simulink model "leader_qball2_mytest"  (R2014a)
settings: Solver=ode1  StartTime=0.0  StopTime=inf  FixedStep=0.002  RelTol=1e-3
InitFcn:
  | QBall_2_Setup
values from neighbouring files (symbols this model uses):
  g = 9.81    [QBall_2_System_Parameters.m]
  joystick_range_max = 0.8    [QBall_2_Setup.m]
  joystick_range_min = 0.5    [QBall_2_Setup.m]
  KdHEIGHT_DOWN = 0.15    [QBall_2_Controller_Design.m]
  KdHEIGHT_UP = 0.15    [QBall_2_Controller_Design.m]
  KdOUTER_PITCH_DOWN = 0.4    [QBall_2_Controller_Design.m]
  KdOUTER_PITCH_UP = 0.6    [QBall_2_Controller_Design.m]
  KdOUTER_ROLL_DOWN = 0.4    [QBall_2_Controller_Design.m]
  KdOUTER_ROLL_UP = 0.4    [QBall_2_Controller_Design.m]
  KdPITCH_DOWN = 0.1    [QBall_2_Controller_Design.m]
  KdPITCH_UP = 0.1    [QBall_2_Controller_Design.m]
  KdROLL_DOWN = 0.1    [QBall_2_Controller_Design.m]
  KdROLL_UP = 0.1    [QBall_2_Controller_Design.m]
  KdYAW_DOWN = 0.32    [QBall_2_Controller_Design.m]
  KdYAW_UP = 0.32    [QBall_2_Controller_Design.m]
  KiHEIGHT_DOWN = 0.35    [QBall_2_Controller_Design.m]
  KiHEIGHT_UP = 0.35    [QBall_2_Controller_Design.m]
  KiOUTER_PITCH_DOWN = 0.08    [QBall_2_Controller_Design.m]
  KiOUTER_PITCH_UP = 0.08    [QBall_2_Controller_Design.m]
  KiOUTER_ROLL_DOWN = 0.08    [QBall_2_Controller_Design.m]
  KiOUTER_ROLL_UP = 0.08    [QBall_2_Controller_Design.m]
  KiPITCH_DOWN = 0.08    [QBall_2_Controller_Design.m]
  KiPITCH_UP = 0.08    [QBall_2_Controller_Design.m]
  KiROLL_DOWN = 0.08    [QBall_2_Controller_Design.m]
  KiROLL_UP = 0.08    [QBall_2_Controller_Design.m]
  KiYAW_DOWN = 0.0    (= 0)    [QBall_2_Controller_Design.m]
  KiYAW_UP = 0.0    (= 0)    [QBall_2_Controller_Design.m]
  KpHEIGHT_DOWN = 0.5    [QBall_2_Controller_Design.m]
  KpHEIGHT_UP = 0.5    [QBall_2_Controller_Design.m]
  KpOUTER_PITCH_DOWN = 0.3    [QBall_2_Controller_Design.m]
  KpOUTER_PITCH_UP = 0.3    [QBall_2_Controller_Design.m]
  KpOUTER_ROLL_DOWN = 0.3    [QBall_2_Controller_Design.m]
  KpOUTER_ROLL_UP = 0.3    [QBall_2_Controller_Design.m]
  KpPITCH_DOWN = 0.5    [QBall_2_Controller_Design.m]
  KpPITCH_UP = 0.5    [QBall_2_Controller_Design.m]
  KpROLL_DOWN = 0.5    [QBall_2_Controller_Design.m]
  KpROLL_UP = 0.5    [QBall_2_Controller_Design.m]
  KpYAW_DOWN = 0.45    [QBall_2_Controller_Design.m]
  KpYAW_UP = 0.45    [QBall_2_Controller_Design.m]
  LIMIT_CMD_PITCH = 5*pi/180    (= 0.0872664625997)    [QBall_2_Controller_Design.m]
  LIMIT_CMD_ROLL = 5*pi/180    (= 0.0872664625997)    [QBall_2_Controller_Design.m]
  LIMIT_MAX_HEIGHT = 2    [QBall_2_Controller_Design.m]
  LIMIT_MAX_X = 1    [QBall_2_Controller_Design.m]
  LIMIT_MAX_Z = 1    [QBall_2_Controller_Design.m]
  LIMIT_MIN_HEIGHT = 0.3    [QBall_2_Controller_Design.m]
  LIMIT_MIN_X = -1    [QBall_2_Controller_Design.m]
  LIMIT_MIN_Z = -1    [QBall_2_Controller_Design.m]
  LIMIT_RATE_HEIGHT = 0.05    [QBall_2_Controller_Design.m]
  LIMIT_RATE_X = 0.15    [QBall_2_Controller_Design.m]
  LIMIT_RATE_YAW = 15*pi/180    (= 0.261799387799)    [QBall_2_Controller_Design.m]
  LIMIT_RATE_Z = 0.15    [QBall_2_Controller_Design.m]
  LIMIT_uCMD_PITCH = 0.5    [QBall_2_Controller_Design.m]
  LIMIT_uCMD_ROLL = 0.5    [QBall_2_Controller_Design.m]
  LIMIT_uCMD_YAW = 0.5    [QBall_2_Controller_Design.m]
  OFFSET_HEIGHT = 0.3    [QBall_2_System_Parameters.m]
  OMEGA_FILTER = 60    [QBall_2_System_Parameters.m]
  TRIM_THROTTLE = M*g/(4*K)    [QBall_2_Controller_Design.m]
  TRIM_U_PITCH = 0.009    [QBall_2_Controller_Design.m]
  TRIM_U_ROLL = -0.0065    [QBall_2_Controller_Design.m]
undefined symbols (not defined in the file or in its folder): DiscIntNeverNeededParam, qc_get_step_size
libraries: simulink x27, quarc_library x27
(part 2 of 3)

== system leader_qball2_mytest/Throttle and height control/Joystick mode throttle ==
  Divide : Product  Inputs=**
  Joystick throttle scaling : Gain  Gain=0.8
  Joystick to Throttle Mapping : MATLAB Function  TreatAsAtomicUnit=on
  height command1 : Constant  Value=joystick_range_min
  height command2 : Constant  Value=joystick_range_max
  throttle joystick : Scope
      settings: YMin=0.45  YMax=1  SaveName=ScopeData26
  throttle : Outport
  wires:
  Divide/1 -> Joystick to Throttle Mapping/1(u)
  [throttle_joystick] -> throttle joystick/1, Divide/2
  [thrust_comp] -> Divide/1
  height command2/1 -> Joystick to Throttle Mapping/3(l2)
  height command1/1 -> Joystick to Throttle Mapping/2(l1)
  Joystick to Throttle Mapping/1(y) -> Joystick throttle scaling/1
  Joystick throttle scaling/1 -> throttle/1

== system leader_qball2_mytest/Throttle and height control/Safety - Active During Emergency Landing: Ramp Throttle CMD down to zero if Sonar Failed  ==
  note: The sonar is only used for an emergency landing if
      | the height mode is set to closed-loop. In joystick
      | height mode, the throttle wind down subsystem is
      | used to reduce the throttle to 0%.
  note: Check if the sonar value is changing.
      | If the sonar value does not change for 1 second
      | we assume the sonar is not connected or is malfunctioning,
      | in which case we want to reduce throttle quickly.
  throttle : Inport
  Limit descent rate : Subsystem
  Logical Operator : Logic  AllPortsSameDT=off  OutDataTypeStr=boolean
  Logical Operator1 : Logic  Operator=NOT  AllPortsSameDT=off  OutDataTypeStr=boolean
  Subsystem : Subsystem
  Switch : Switch  Threshold=0.5
  land w/ sonar : Scope
      settings: YMin=-0.2  YMax=1.2  SaveName=ScopeData25
  Out1 : Outport
  wires:
  Limit descent rate/1(throttle wind down) -> Switch/1
  Logical Operator/1 -> Switch/2
  Switch/1 -> Out1/1
  [land] -> Logical Operator/1, Limit descent rate/2(land)
  throttle/1 -> Switch/3, Limit descent rate/1(throttle)
  Subsystem/1(land with sonar) -> land w/ sonar/1, Logical Operator1/1
  Logical Operator1/1 -> Logical Operator/2

== system leader_qball2_mytest/Throttle and height control/height control ==
  height command : Inport
  Manual Switch : ManualSwitch  CurrentSetting=0
  Safety - Emergency Landing (Set Height Ref CMD to zero) : Subsystem
  Saturation3 : Saturate  UpperLimit=2  LowerLimit=0
  sigmoid1 : Subsystem
  sonar controller : Subsystem
  sonar height : Subsystem
  throttle : Outport
  tag scope: h_cmd=global
  wires:
  sonar controller/1(control_action) -> throttle/1
  sigmoid1/1(height_cmd) -> sonar controller/1(cmd), [h_cmd]
  sonar height/1(sonar (adjusted)) -> Saturation3/1
  Safety - Emergency Landing (Set Height Ref CMD to zero)/1(Out1) -> sigmoid1/1(cmd)
  height command/1 -> Safety - Emergency Landing (Set Height Ref CMD to zero)/1(In1)
  Saturation3/1 -> Manual Switch/1
  Manual Switch/1 -> sigmoid1/2(height), sonar controller/2(height)
  [height_above_ground] -> Manual Switch/2

== system leader_qball2_mytest/Control signal mixing/Safety - Motor Shutoff if: - Roll//Pitch Data Runaway (> 40 deg) - Initial 3 second of execution for motor initialization/Enabled Subsystem ==
  Enable : EnablePort
  Constant : Constant  Value=0
  Out1 : Outport  InitialOutput=1
  wires:
  Constant/1 -> Out1/1

== system leader_qball2_mytest/Control signal mixing/Safety - Motor Shutoff if: - Roll//Pitch Data Runaway (> 40 deg) - Initial 3 second of execution for motor initialization/throttle enable ==
  note: This check is obsolete - originally for protecting against invalid PWM command to ESC (for QBall-X4).
  Compare To Constant : simulink/Logic and Bit Operations/Compare To Constant  relop=<=  const=0.0525  OutDataTypeStr=uint8  ZeroCross=off
  Constant2 : Constant  Value=2
  Enabled Subsystem : Subsystem  TreatAsAtomicUnit=on
  Logical Operator1 : Logic  Operator=NOT  AllPortsSameDT=off  OutDataTypeStr=boolean
  en : Outport
  wires:
  [throttle_cmd] -> Compare To Constant/1
  Compare To Constant/1 -> Enabled Subsystem/Enable
  Enabled Subsystem/1(timeout) -> Logical Operator1/1
  Logical Operator1/1 -> en/1
  Constant2/1 -> Enabled Subsystem/1(timeout limit)

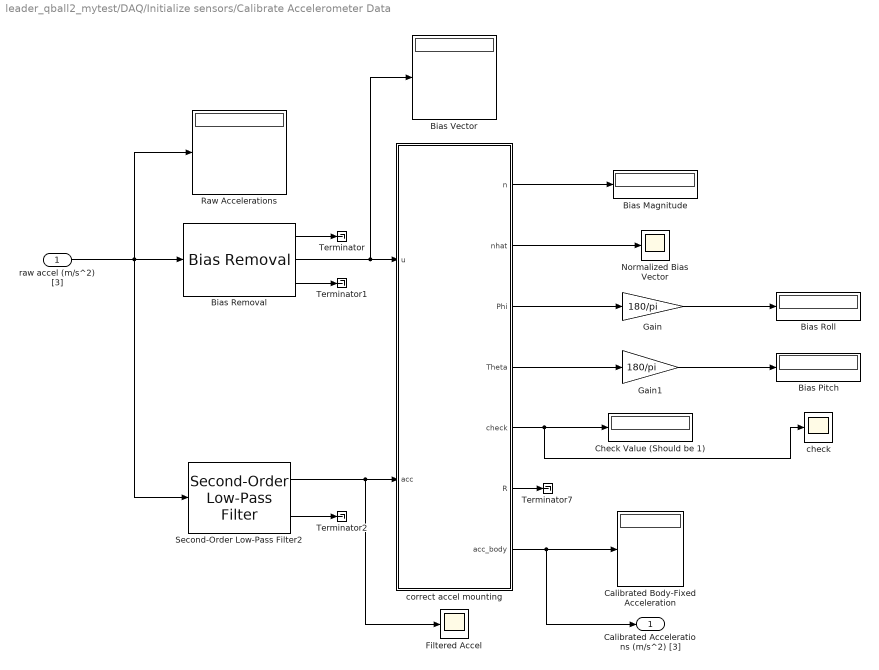
== system leader_qball2_mytest/DAQ/Initialize sensors/Calibrate Accelerometer Data ==
  raw accel (m/s^2) [3] : Inport
  Bias Magnitude : Display
      settings: Decimation=100
  Bias Pitch : Display
      settings: Decimation=100
  Bias Removal : quarc_library/Discrete/Bias Removal  start_time=0  end_time=TIMEOUT_CALIB  switch_id=0  sample_time=qc_get_step_size
  Bias Roll : Display
      settings: Decimation=100
  Bias Vector : Display
      settings: Decimation=100
  Calibrated Body-Fixed Acceleration : Display
      settings: Decimation=100
  Check Value (Should be 1) : Display
      settings: Decimation=100
  Filtered Accel : Scope
      settings: YMin=-200  YMax=200  SaveName=ScopeData42
  Gain : Gain  Gain=180/pi
  Gain1 : Gain  Gain=180/pi
  Normalized Bias Vector : Scope
  Raw Accelerations : Display
      settings: Decimation=100
  Second-Order Low-Pass Filter2 : quarc_library/Continuous/Second-Order Low-Pass Filter  params_source=Internal (dialog parameters)  input_width=OMEGA_FILTER  input_zeta=1  input_init=0
  Terminator{,1..2,7} (4 alike) : Terminator
  check : Scope
      settings: YMin=0.95  YMax=1.05  SaveName=ScopeData12
  correct accel mounting : MATLAB Function  TreatAsAtomicUnit=on
  Calibrated Accelerations (m/s^2) [3] : Outport
  wires:
  Bias Removal/2 -> Bias Vector/1, correct accel mounting/1(u)
  correct accel mounting/1(n) -> Bias Magnitude/1
  correct accel mounting/2(nhat) -> Normalized Bias Vector/1
  correct accel mounting/3(Phi) -> Gain/1
  correct accel mounting/4(Theta) -> Gain1/1
  Gain/1 -> Bias Roll/1
  Gain1/1 -> Bias Pitch/1
  correct accel mounting/5(check) -> check/1, Check Value (Should be 1)/1
  Bias Removal/1 -> Terminator/1
  Bias Removal/3 -> Terminator1/1
  correct accel mounting/6(R) -> Terminator7/1
  correct accel mounting/7(acc_body) -> Calibrated Accelerations (m/s^2) [3]/1, Calibrated Body-Fixed Acceleration/1
  raw accel (m/s^2) [3]/1 -> Raw Accelerations/1, Second-Order Low-Pass Filter2/1, Bias Removal/1
  Second-Order Low-Pass Filter2/1 -> Filtered Accel/1, correct accel mounting/2(acc)
  Second-Order Low-Pass Filter2/2 -> Terminator2/1

== system leader_qball2_mytest/DAQ/Initialize sensors/Calibrate accelerometer (Obsolete) ==
  In1 : Inport
  Calibration time (s) : Constant
  Clock : Clock
  Demux : Demux  Outputs=3
  Demux1 : Demux  Outputs=3
  Enabled Moving Average : quarc_library/Discrete/Enabled Moving Average  enable_state=reset  sample_time=qc_get_step_size
  Mux : Mux  Inputs=2
  Relational Operator : RelationalOperator  Operator=<  OutDataTypeStr=boolean
  Sum : Sum  Inputs=|+-
  Sum1 : Sum  Inputs=|+-
  Terminator{,1..3} (4 alike) : Terminator
  accel calibrated : Scope
      settings: YMin=-13  SaveName=ScopeData17
  accels offset : Scope
      settings: YMin=-13  SaveName=ScopeData16
  initial accel : Constant  Value=[0 0 -9.81]
  Out1 : Outport
  wires:
  In1/1 -> Sum1/1, Sum/1, Demux/1
  Clock/1 -> Relational Operator/1
  Calibration time (s)/1 -> Relational Operator/2
  Relational Operator/1 -> Enabled Moving Average/Enable
  Sum/1 -> Out1/1, Demux1/1
  initial accel/1 -> Sum1/2
  Sum1/1 -> Enabled Moving Average/1
  Enabled Moving Average/1 -> Sum/2, accels offset/1
  Demux/2 -> Mux/1
  Demux1/2 -> Mux/2
  Mux/1 -> accel calibrated/1
  Demux/1 -> Terminator/1
  Demux/3 -> Terminator1/1
  Demux1/1 -> Terminator2/1
  Demux1/3 -> Terminator3/1

== system leader_qball2_mytest/DAQ/Initialize sensors/Nonlinear Limit (Reject Spikes) ==
  u : Inport
  Constant : Constant  Value=0.5
  Embedded MATLAB Function : MATLAB Function  TreatAsAtomicUnit=on
  Memory : Memory
  y : Outport
  wires:
  Embedded MATLAB Function/1(y) -> Memory/1, y/1
  Memory/1 -> Embedded MATLAB Function/2(x)
  u/1 -> Embedded MATLAB Function/1(u)
  Constant/1 -> Embedded MATLAB Function/3(threshold)

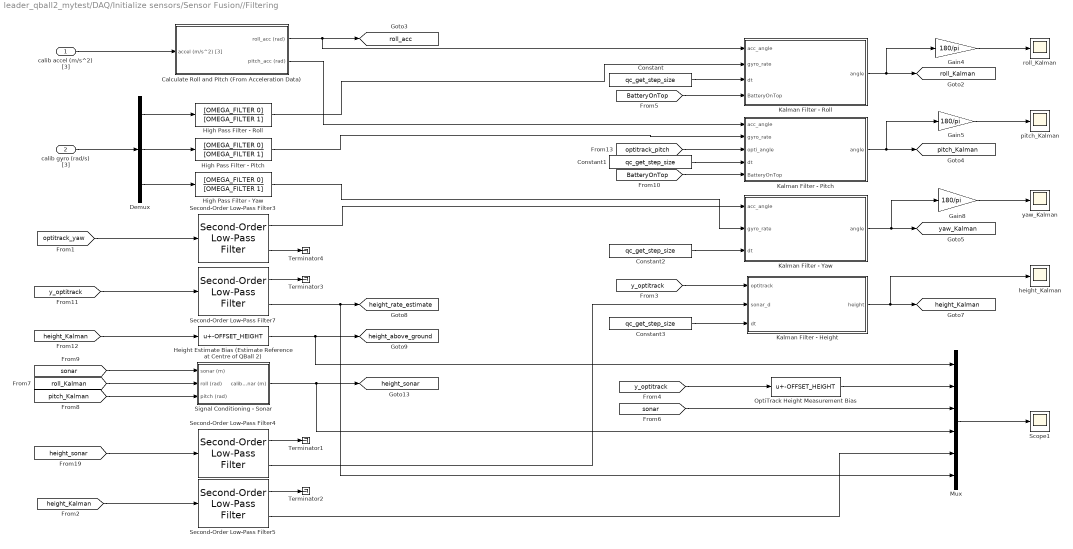
== system leader_qball2_mytest/DAQ/Initialize sensors/Sensor Fusion//Filtering ==
  calib accel (m/s^2) [3] : Inport
  calib gyro (rad/s) [3] : Inport  Port=2
  Calculate Roll and Pitch (From Acceleration Data) : Subsystem
  Constant{,1..3} (4 alike) : Constant  Value=qc_get_step_size
  Demux : Demux  Outputs=3
  Gain4 : Gain  Gain=180/pi
  Gain5 : Gain  Gain=180/pi
  Gain8 : Gain  Gain=180/pi
  "Height Estimate Bias (Estimate Reference at Centre of QBall 2) " : Bias  Bias=-OFFSET_HEIGHT
  High Pass Filter - Pitch : TransferFcn  Numerator=[OMEGA_FILTER 0]  Denominator=[OMEGA_FILTER 1]
  High Pass Filter - Roll : TransferFcn  Numerator=[OMEGA_FILTER 0]  Denominator=[OMEGA_FILTER 1]
  High Pass Filter - Yaw : TransferFcn  Numerator=[OMEGA_FILTER 0]  Denominator=[OMEGA_FILTER 1]
  Kalman Filter - Height : MATLAB Function  TreatAsAtomicUnit=on
  Kalman Filter - Pitch : MATLAB Function  TreatAsAtomicUnit=on
  Kalman Filter - Roll : MATLAB Function  TreatAsAtomicUnit=on
  Kalman Filter - Yaw : MATLAB Function  TreatAsAtomicUnit=on
  Mux : Mux  Inputs=6
  OptiTrack Height Measurement Bias : Bias  Bias=-OFFSET_HEIGHT
  Scope1 : Scope
      settings: YMin=-1.5  YMax=1.5  SaveName=ScopeData53
  Second-Order Low-Pass Filter3 : quarc_library/Continuous/Second-Order Low-Pass Filter  params_source=Internal (dialog parameters)  input_width=OMEGA_FILTER  input_zeta=1  input_init=0
  Second-Order Low-Pass Filter4 : quarc_library/Continuous/Second-Order Low-Pass Filter  params_source=Internal (dialog parameters)  input_width=OMEGA_DIFF  input_zeta=1  input_init=0
  Second-Order Low-Pass Filter5 : quarc_library/Continuous/Second-Order Low-Pass Filter  params_source=Internal (dialog parameters)  input_width=OMEGA_DIFF  input_zeta=1  input_init=0
  Second-Order Low-Pass Filter7 : quarc_library/Continuous/Second-Order Low-Pass Filter  params_source=Internal (dialog parameters)  input_width=OMEGA_DIFF  input_zeta=1  input_init=0
  Signal Conditioning - Sonar : Subsystem
  Terminator{1..4} (4 alike) : Terminator
  height_Kalman : Scope
      settings: YMin=17.282  YMax=17.292  SaveName=ScopeData52
  pitch_Kalman : Scope
      settings: TimeRange=10  YMin=-45  YMax=60  SaveName=ScopeData39
  roll_Kalman : Scope
      settings: YMin=-100  YMax=100  SaveName=ScopeData36
  yaw_Kalman : Scope
      settings: YMin=-70  YMax=110  SaveName=ScopeData47
  tag scope: height_Kalman=global, height_above_ground=global, height_rate_estimate=global, height_sonar=global, pitch_Kalman=global, roll_Kalman=global, roll_acc=global, yaw_Kalman=global
  wires:
  Kalman Filter - Roll/1(angle) -> [roll_Kalman], Gain4/1
  Demux/2 -> High Pass Filter - Pitch/1
  Constant/1 -> Kalman Filter - Roll/3(dt)
  Constant1/1 -> Kalman Filter - Pitch/4(dt)
  Kalman Filter - Pitch/1(angle) -> [pitch_Kalman], Gain5/1
  Gain5/1 -> pitch_Kalman/1
  Demux/3 -> High Pass Filter - Yaw/1
  Gain4/1 -> roll_Kalman/1
  calib gyro (rad/s) [3]/1 -> Demux/1
  Demux/1 -> High Pass Filter - Roll/1
  High Pass Filter - Roll/1 -> Kalman Filter - Roll/2(gyro_rate)
  [optitrack_yaw] -> Second-Order Low-Pass Filter3/1
  Second-Order Low-Pass Filter3/1 -> Kalman Filter - Yaw/1(acc_angle)
  High Pass Filter - Yaw/1 -> Kalman Filter - Yaw/2(gyro_rate)
  Constant2/1 -> Kalman Filter - Yaw/3(dt)
  Kalman Filter - Yaw/1(angle) -> [yaw_Kalman], Gain8/1
  Gain8/1 -> yaw_Kalman/1
  Constant3/1 -> Kalman Filter - Height/3(dt)
  Kalman Filter - Height/1(height) -> height_Kalman/1, [height_Kalman]
  Mux/1 -> Scope1/1
  Second-Order Low-Pass Filter4/2 -> Kalman Filter - Height/2(sonar_d)
  [y_optitrack] -> OptiTrack Height Measurement Bias/1
  [sonar] -> Mux/3
  OptiTrack Height Measurement Bias/1 -> Mux/2
  [y_optitrack] -> Kalman Filter - Height/1(optitrack)
  [height_Kalman] -> Second-Order Low-Pass Filter5/1
  Second-Order Low-Pass Filter5/2 -> Mux/5
  [y_optitrack] -> Second-Order Low-Pass Filter7/1
  Second-Order Low-Pass Filter7/2 -> Mux/6, [height_rate_estimate]
  [height_Kalman] -> "Height Estimate Bias (Estimate Reference at Centre of QBall 2) "/1
  "Height Estimate Bias (Estimate Reference at Centre of QBall 2) "/1 -> Mux/1, [height_above_ground]
  calib accel (m/s^2) [3]/1 -> Calculate Roll and Pitch (From Acceleration Data)/1(accel (m/s^2) [3])
  Calculate Roll and Pitch (From Acceleration Data)/1(roll_acc (rad)) -> Kalman Filter - Roll/1(acc_angle), [roll_acc]
  Calculate Roll and Pitch (From Acceleration Data)/2(pitch_acc (rad)) -> Kalman Filter - Pitch/1(acc_angle)
  Second-Order Low-Pass Filter3/2 -> Terminator4/1
  Second-Order Low-Pass Filter7/1 -> Terminator3/1
  [roll_Kalman] -> Signal Conditioning - Sonar/2(roll (rad))
  [pitch_Kalman] -> Signal Conditioning - Sonar/3(pitch (rad))
  [sonar] -> Signal Conditioning - Sonar/1(sonar (m))
  Signal Conditioning - Sonar/1(calib sonar (m)) -> Mux/4, [height_sonar]
  [height_sonar] -> Second-Order Low-Pass Filter4/1
  Second-Order Low-Pass Filter4/1 -> Terminator1/1
  Second-Order Low-Pass Filter5/1 -> Terminator2/1
  High Pass Filter - Pitch/1 -> Kalman Filter - Pitch/2(gyro_rate)
  [BatteryOnTop] -> Kalman Filter - Roll/4(BatteryOnTop)
  [BatteryOnTop] -> Kalman Filter - Pitch/5(BatteryOnTop)
  [optitrack_pitch] -> Kalman Filter - Pitch/3(opti_angle)

== system leader_qball2_mytest/DAQ/Initialize sensors/Zero gyro ==
  In1 : Inport
  Calibration time (s) : Constant
  Clock : Clock
  Enabled Moving Average : quarc_library/Discrete/Enabled Moving Average  enable_state=reset  sample_time=qc_get_step_size
  Relational Operator : RelationalOperator  Operator=<  OutDataTypeStr=boolean
  Sum : Sum  Inputs=|+-
  Out1 : Outport
  wires:
  Sum/1 -> Out1/1
  Relational Operator/1 -> Enabled Moving Average/Enable
  Calibration time (s)/1 -> Relational Operator/2
  Clock/1 -> Relational Operator/1
  Enabled Moving Average/1 -> Sum/2
  In1/1 -> Sum/1, Enabled Moving Average/1

== system leader_qball2_mytest/Data from host/rcvd packet monitoring/spike detection ==
  In1 : Inport
  Abs : Abs
  Compare To Constant : simulink/Logic and Bit Operations/Compare To Constant  relop=>=  const=100  OutDataTypeStr=boolean  ZeroCross=off
  Logical Operator4 : Logic  Operator=OR  Inputs=1  AllPortsSameDT=off  OutDataTypeStr=boolean
  Show Message on Host1 : quarc_library/Sinks/Error Handling/Show Message on Host  message_type=Fixed error message  message_icon=Warning  message=Spike detected!
      settings: AttributesFormatString="\"%<message>\""
  wires:
  Abs/1 -> Compare To Constant/1
  Compare To Constant/1 -> Logical Operator4/1
  Logical Operator4/1 -> Show Message on Host1/1
  In1/1 -> Abs/1

== system leader_qball2_mytest/Data from host/timeout safety/Enabled Subsystem ==
  timeout limit : Inport
  Enable : EnablePort  StatesWhenEnabling=reset
  Constant : Constant  SampleTime=qc_get_step_size
  Discrete-Time Integrator : DiscreteIntegrator  SampleTime=-1  ICPrevOutput=DiscIntNeverNeededParam  ICPrevScaledInput=DiscIntNeverNeededParam
  Relational Operator : RelationalOperator  OutDataTypeStr=boolean
  timeout : Outport  OutputWhenDisabled=reset  InitialOutput=[0]
  wires:
  Relational Operator/1 -> timeout/1
  timeout limit/1 -> Relational Operator/2
  Discrete-Time Integrator/1 -> Relational Operator/1
  Constant/1 -> Discrete-Time Integrator/1

== system leader_qball2_mytest/Data from host/timeout safety/Enabled Subsystem1 ==
  timeout limit : Inport
  Enable : EnablePort  StatesWhenEnabling=reset
  Constant : Constant  SampleTime=qc_get_step_size
  Discrete-Time Integrator : DiscreteIntegrator  SampleTime=-1  ICPrevOutput=DiscIntNeverNeededParam  ICPrevScaledInput=DiscIntNeverNeededParam
  Relational Operator : RelationalOperator  OutDataTypeStr=boolean
  timeout : Outport  OutputWhenDisabled=reset  InitialOutput=[0]
  wires:
  Relational Operator/1 -> timeout/1
  timeout limit/1 -> Relational Operator/2
  Discrete-Time Integrator/1 -> Relational Operator/1
  Constant/1 -> Discrete-Time Integrator/1

== system leader_qball2_mytest/Data from host/timeout safety/Enabled Subsystem2 ==
  Enable : EnablePort
  Constant : Constant
  Out1 : Outport  InitialOutput=0
  wires:
  Constant/1 -> Out1/1

== system leader_qball2_mytest/Data from host/timeout safety/Enabled Subsystem Latch Output High ==
  Enable : EnablePort
  Constant : Constant
  Out1 : Outport  InitialOutput=0
  wires:
  Constant/1 -> Out1/1

== system leader_qball2_mytest/Pitch Controller/Subsystem/OT pos control ==
  Compare To Constant : simulink/Logic and Bit Operations/Compare To Constant  relop=>  const=0.4*0  OutDataTypeStr=uint8  ZeroCross=off
  Mux1 : Mux  Inputs=2
  Orig v. adjusted pitch : Scope
      settings: YMin=-0.1  YMax=0.12  SaveName=ScopeData21
  Product : Product  RndMeth=Zero
  Sum2 : Sum  Inputs=+-
  adjust_for_heading : Subsystem
  rate limitted control : Subsystem
  pitch cmd : Outport
  tag scope: pitch_workspace_frame=global
  wires:
  rate limitted control/1(Pitch Ref CMD (rad)) -> Product/1, [pitch_workspace_frame]
  Sum2/1 -> rate limitted control/1(error)
  Product/1 -> Mux1/1, adjust_for_heading/1(original)
  Compare To Constant/1 -> Product/2
  [y_optitrack] -> Compare To Constant/1
  Mux1/1 -> Orig v. adjusted pitch/1
  adjust_for_heading/1(heading_adjusted pitch) -> Mux1/2, pitch cmd/1
  [z_optitrack] -> Sum2/2
  [z_pos_cmd] -> Sum2/1

== system leader_qball2_mytest/Pitch Controller/Subsystem/Safety - Emergency Landing Zero Ref CMD ==
  In1 : Inport
  Constant : Constant  Value=0
  Enabled Subsystem : Subsystem  TreatAsAtomicUnit=on
  Switch : Switch  Threshold=0.5
  Out1 : Outport
  wires:
  [land] -> Enabled Subsystem/Enable
  Constant/1 -> Switch/1
  Enabled Subsystem/1(Out1) -> Switch/2
  In1/1 -> Switch/3
  Switch/1 -> Out1/1

== system leader_qball2_mytest/Roll Controller/Subsystem/OT pos control ==
  Compare To Constant : simulink/Logic and Bit Operations/Compare To Constant  relop=>  const=0.4*0  OutDataTypeStr=uint8  ZeroCross=off
  Mux1 : Mux  Inputs=2
  Mux2 : Mux  Inputs=2
  Orig v. adjusted roll : Scope
      settings: YMin=-0.12  YMax=0.09  SaveName=ScopeData22
  Product : Product  RndMeth=Zero
  Sum1 : Sum  Inputs=+-
  X_cmd and X_meas : Scope
      settings: YMin=0  YMax=0.11  SaveName=ScopeData11
  adjust_for_heading : Subsystem
  rate limitted control : Subsystem
  roll cmd : Outport
  tag scope: roll_workspace_frame=global
  wires:
  rate limitted control/1(Roll Ref CMD (rad)) -> Product/1, [roll_workspace_frame]
  Sum1/1 -> rate limitted control/1(error)
  Product/1 -> Mux1/1, adjust_for_heading/1(original)
  Compare To Constant/1 -> Product/2
  [y_optitrack] -> Compare To Constant/1
  Mux1/1 -> Orig v. adjusted roll/1
  adjust_for_heading/1(heading_adjusted roll) -> Mux1/2, roll cmd/1
  [x_optitrack] -> Sum1/2, Mux2/2
  [x_pos_cmd] -> Sum1/1, Mux2/1
  Mux2/1 -> X_cmd and X_meas/1

== system leader_qball2_mytest/Roll Controller/Subsystem/Safety - Emergency Landing Zero Ref CMD ==
  In1 : Inport
  Constant : Constant  Value=0
  Enabled Subsystem : Subsystem  TreatAsAtomicUnit=on
  Switch : Switch  Threshold=0.5
  Out1 : Outport
  wires:
  Switch/1 -> Out1/1
  In1/1 -> Switch/3
  Enabled Subsystem/1(Out1) -> Switch/2
  Constant/1 -> Switch/1
  [land] -> Enabled Subsystem/Enable

== system leader_qball2_mytest/Throttle and height control/Safety - Active During Emergency Landing: Ramp Throttle CMD down to zero if Sonar Failed /Limit descent rate ==
  throttle : Inport
  land : Inport  Port=2
  Constant1 : Constant  Value=0
  Terminator : Terminator
  Terminator1 : Terminator
  Terminator2 : Terminator
  Triggered Sigmoid : quarc_library/Sources/Sigmoids/Triggered Sigmoid  params_source=Internal (dialog parameters)  max_velocity=0.04  max_acceleration=1000*20  hold_off=0.5  output_sample_time=qc_get_step_size  trigger=rising
  land throttle target : Constant  Value=0
  throttle wind down : Outport
  wires:
  Triggered Sigmoid/1 -> throttle wind down/1
  land throttle target/1 -> Triggered Sigmoid/4
  Constant1/1 -> Triggered Sigmoid/3
  throttle/1 -> Triggered Sigmoid/2
  land/1 -> Triggered Sigmoid/1
  Triggered Sigmoid/2 -> Terminator/1
  Triggered Sigmoid/3 -> Terminator1/1
  Triggered Sigmoid/4 -> Terminator2/1

== system leader_qball2_mytest/Throttle and height control/Safety - Active During Emergency Landing: Ramp Throttle CMD down to zero if Sonar Failed /Subsystem ==
  Compare To Constant : simulink/Logic and Bit Operations/Compare To Constant  relop===  const=1  OutDataTypeStr=uint8
  Compare To Zero : simulink/Logic and Bit Operations/Compare To Zero  relop===  OutDataTypeStr=boolean  ZeroCross=off
  Constant1 : Constant  Value=0
  Constant2 : Constant  Value=5
  Derivative : Derivative
  Enabled Subsystem1 : Subsystem  TreatAsAtomicUnit=on
  Logical Operator : Logic  AllPortsSameDT=off  OutDataTypeStr=boolean
  Logical Operator3 : Logic  Operator=NOT  AllPortsSameDT=off  OutDataTypeStr=boolean
  Manual Switch : ManualSwitch
  land with sonar : Outport
  wires:
  Logical Operator3/1 -> Logical Operator/1
  Compare To Constant/1 -> Logical Operator/2
  [height_mode] -> Compare To Constant/1
  Logical Operator/1 -> land with sonar/1
  Enabled Subsystem1/1(timeout) -> Logical Operator3/1
  Constant1/1 -> Manual Switch/2
  [sonar] -> Manual Switch/1
  Manual Switch/1 -> Derivative/1
  Constant2/1 -> Enabled Subsystem1/1(timeout limit)
  Compare To Zero/1 -> Enabled Subsystem1/Enable
  Derivative/1 -> Compare To Zero/1

== system leader_qball2_mytest/Throttle and height control/height control/Safety - Emergency Landing (Set Height Ref CMD to zero) ==
  In1 : Inport
  Constant : Constant  Value=0
  Enabled Subsystem : Subsystem  TreatAsAtomicUnit=on
  Switch : Switch  Threshold=0.5
  Out1 : Outport
  wires:
  Constant/1 -> Switch/1
  [land] -> Enabled Subsystem/Enable
  Enabled Subsystem/1(Out1) -> Switch/2
  In1/1 -> Switch/3
  Switch/1 -> Out1/1

== system leader_qball2_mytest/Throttle and height control/height control/sigmoid1 ==
  cmd : Inport
  height : Inport  Port=2
  Continuous Sigmoid : quarc_library/Sources/Sigmoids/Continuous Sigmoid  params_source=External (input ports)  max_velocity=2  max_acceleration=10  initial_position=0  initial_velocity=0  hold_off=0.5  input_sample_time=-1  output_sample_time=qc_get_step_size
  Terminator : Terminator
  Terminator1 : Terminator
  Terminator2 : Terminator
  arm height command : Subsystem  TreatAsAtomicUnit=on
  sigmoid limits : Subsystem
  height_cmd : Outport
  wires:
  Continuous Sigmoid/4 -> Terminator2/1
  Continuous Sigmoid/3 -> Terminator1/1
  Continuous Sigmoid/2 -> Terminator/1
  arm height command/1(Out1) -> Continuous Sigmoid/1
  cmd/1 -> arm height command/1(In1), sigmoid limits/1(height cmd)
  sigmoid limits/1(vmax) -> Continuous Sigmoid/2
  sigmoid limits/2(amax) -> Continuous Sigmoid/3
  [armed] -> arm height command/Enable
  height/1 -> sigmoid limits/2(height)
  Continuous Sigmoid/1 -> height_cmd/1

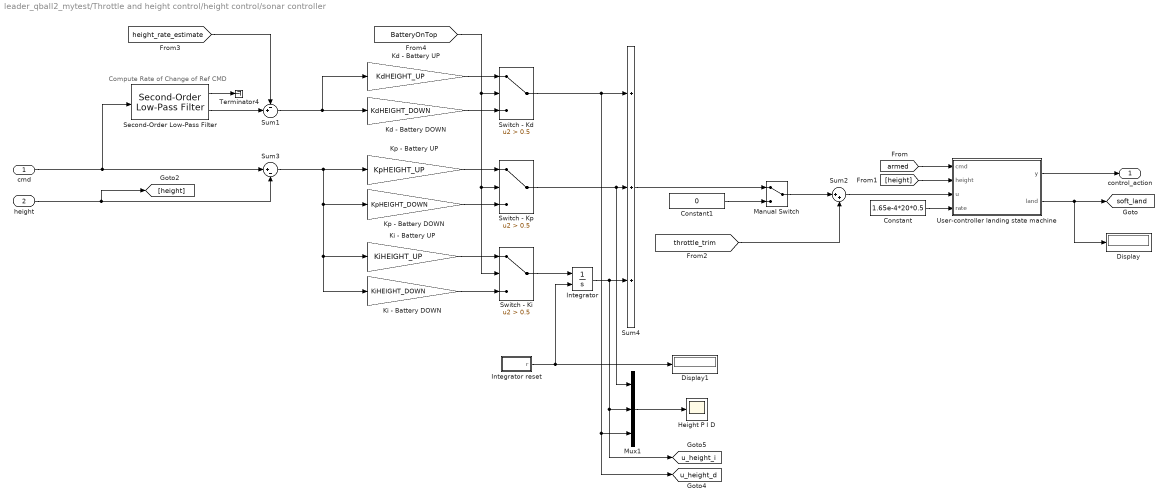
== system leader_qball2_mytest/Throttle and height control/height control/sonar controller ==
  note: Compute Rate of Change of Ref CMD
  cmd : Inport
  height : Inport  Port=2
  Constant : Constant  Value=1.65e-4*20*0.5
  Constant1 : Constant  Value=0
  Display : Display
      settings: Decimation=100
  Display1 : Display
      settings: Decimation=100
  Height P I D : Scope
      settings: YMin=-0.065  YMax=0.04  SaveName=ScopeData37
  Integrator : Integrator  ExternalReset=level  LimitOutput=on  UpperSaturationLimit=1  LowerSaturationLimit=0
  Integrator reset : Subsystem
  Kd - Battery DOWN : Gain  Gain=KdHEIGHT_DOWN
  Kd - Battery UP : Gain  Gain=KdHEIGHT_UP
  Ki - Battery DOWN : Gain  Gain=KiHEIGHT_DOWN
  Ki - Battery UP : Gain  Gain=KiHEIGHT_UP
  Kp - Battery DOWN : Gain  Gain=KpHEIGHT_DOWN
  Kp - Battery UP : Gain  Gain=KpHEIGHT_UP
  Manual Switch : ManualSwitch
  Mux1 : Mux  Inputs=3
  Second-Order Low-Pass Filter : quarc_library/Continuous/Second-Order Low-Pass Filter  params_source=Internal (dialog parameters)  input_width=OMEGA_DIFF  input_zeta=1  input_init=0
  Sum1 : Sum  Inputs=-+|
  Sum2 : Sum  Inputs=|++
  Sum3 : Sum  Inputs=|+-
  Sum4 : Sum  Inputs=+++
  Switch - Kd : Switch  Criteria=u2 > Threshold  Threshold=0.5
  Switch - Ki : Switch  Criteria=u2 > Threshold  Threshold=0.5
  Switch - Kp : Switch  Criteria=u2 > Threshold  Threshold=0.5
  Terminator4 : Terminator
  User-controller landing state machine : MATLAB Function  TreatAsAtomicUnit=on
  control_action : Outport
  tag scope: soft_land=global, u_height_d=global, u_height_i=global
  wires:
  Constant/1 -> User-controller landing state machine/4(rate)
  User-controller landing state machine/2(land) -> [soft_land], Display/1
  [height] -> User-controller landing state machine/2(height)
  [armed] -> User-controller landing state machine/1(cmd)
  User-controller landing state machine/1(y) -> control_action/1
  Mux1/1 -> Height P I D/1
  height/1 -> Sum3/2, [height]
  cmd/1 -> Sum3/1, Second-Order Low-Pass Filter/1
  Sum3/1 -> Kp - Battery UP/1, Ki - Battery UP/1, Ki - Battery DOWN/1, Kp - Battery DOWN/1
  Integrator reset/1(r) -> Display1/1, Integrator/2
  Integrator/1 -> [u_height_i], Mux1/2, Sum4/3
  Sum1/1 -> Kd - Battery DOWN/1, Kd - Battery UP/1
  Sum4/1 -> Manual Switch/1
  Constant1/1 -> Manual Switch/2
  Manual Switch/1 -> Sum2/1
  [throttle_trim] -> Sum2/2
  Sum2/1 -> User-controller landing state machine/3(u)
  Second-Order Low-Pass Filter/1 -> Terminator4/1
  Kd - Battery UP/1 -> Switch - Kd/1
  Kd - Battery DOWN/1 -> Switch - Kd/3
  [BatteryOnTop] -> Switch - Kp/2, Switch - Ki/2, Switch - Kd/2
  Switch - Kd/1 -> Mux1/3, [u_height_d], Sum4/1
  Kp - Battery UP/1 -> Switch - Kp/1
  Kp - Battery DOWN/1 -> Switch - Kp/3
  Switch - Kp/1 -> Mux1/1, Sum4/2
  [height_rate_estimate] -> Sum1/1
  Second-Order Low-Pass Filter/2 -> Sum1/2
  Ki - Battery DOWN/1 -> Switch - Ki/3
  Switch - Ki/1 -> Integrator/1
  Ki - Battery UP/1 -> Switch - Ki/1

== system leader_qball2_mytest/Throttle and height control/height control/sonar height ==
  Product : Product  Inputs=3  RndMeth=Zero
  Trigonometric Function : Trigonometry  Operator=cos
  Trigonometric Function2 : Trigonometry  Operator=cos
  sonar (adjusted) : Outport
  wires:
  Trigonometric Function2/1 -> Product/1
  [pitch_Kalman] -> Trigonometric Function2/1
  Trigonometric Function/1 -> Product/2
  Product/1 -> sonar (adjusted)/1
  [roll_Kalman] -> Trigonometric Function/1
  [sonar] -> Product/3

== system leader_qball2_mytest/Control signal mixing/Safety - Motor Shutoff if: - Roll//Pitch Data Runaway (> 40 deg) - Initial 3 second of execution for motor initialization/throttle enable/Enabled Subsystem ==
  timeout limit : Inport
  Enable : EnablePort  StatesWhenEnabling=reset
  Constant : Constant  SampleTime=qc_get_step_size
  Discrete-Time Integrator : DiscreteIntegrator  SampleTime=-1  ICPrevOutput=DiscIntNeverNeededParam  ICPrevScaledInput=DiscIntNeverNeededParam
  Relational Operator : RelationalOperator  OutDataTypeStr=boolean
  timeout : Outport  OutputWhenDisabled=reset  InitialOutput=[0]
  wires:
  Constant/1 -> Discrete-Time Integrator/1
  Discrete-Time Integrator/1 -> Relational Operator/1
  timeout limit/1 -> Relational Operator/2
  Relational Operator/1 -> timeout/1

== system leader_qball2_mytest/DAQ/Initialize sensors/Sensor Fusion//Filtering/Calculate Roll and Pitch (From Acceleration Data) ==
  accel (m/s^2) [3] : Inport
  Gain{1..2,6..7} (4 alike) : Gain  Gain=180/pi
  calc_roll_pitch : MATLAB Function  TreatAsAtomicUnit=on
  calc_roll_pitch_asin : MATLAB Function  TreatAsAtomicUnit=on
  pitch_acc : Scope
      settings: YMin=-60  YMax=45  SaveName=ScopeData28
  pitch_acc_asin : Scope
      settings: YMin=-10  YMax=27.5  SaveName=ScopeData43
  roll_acc : Scope
      settings: YMin=-200  YMax=200  SaveName=ScopeData20
  roll_acc_asin : Scope
      settings: TimeRange=10  YMin=-10  YMax=27.5  SaveName=ScopeData29
  roll_acc (rad) : Outport
  pitch_acc (rad) : Outport  Port=2
  wires:
  accel (m/s^2) [3]/1 -> calc_roll_pitch_asin/1(acc_body), calc_roll_pitch/1(acc_body)
  calc_roll_pitch/1(roll_acc) -> Gain2/1, roll_acc (rad)/1
  calc_roll_pitch/2(pitch_acc) -> Gain1/1, pitch_acc (rad)/1
  Gain2/1 -> roll_acc/1
  Gain1/1 -> pitch_acc/1
  calc_roll_pitch_asin/1(roll_acc) -> Gain6/1
  Gain6/1 -> roll_acc_asin/1
  calc_roll_pitch_asin/2(pitch_acc) -> Gain7/1
  Gain7/1 -> pitch_acc_asin/1

== system leader_qball2_mytest/DAQ/Initialize sensors/Sensor Fusion//Filtering/Signal Conditioning - Sonar ==
  note: Correct for Roll and Pitch
  note: "Smooth" out the Sonar data
  note: Resample the 10Hz Sonar Data
  sonar (m) : Inport
  roll (rad) : Inport  Port=2
  pitch (rad) : Inport  Port=3
  FOH1 : Subsystem  mask{Ts=0.1}
      mask prompts: Ts "Sample Time"
  Product : Product  Inputs=3  RndMeth=Zero
  Rate Transition : RateTransition
  Sampler : Subsystem  mask{Ts=0.1}
      mask prompts: Ts "Sample Time"
  Trigonometric Function : Trigonometry  Operator=cos
  Trigonometric Function2 : Trigonometry  Operator=cos
  calib sonar (m) : Outport
  wires:
  Sampler/1(Out1) -> Rate Transition/1
  Rate Transition/1 -> FOH1/1(Input)
  sonar (m)/1 -> Sampler/1(In1)
  FOH1/1(Output) -> Product/1
  Trigonometric Function2/1 -> Product/2
  roll (rad)/1 -> Trigonometric Function2/1
  pitch (rad)/1 -> Trigonometric Function/1
  Trigonometric Function/1 -> Product/3
  Product/1 -> calib sonar (m)/1

== system leader_qball2_mytest/Pitch Controller/Subsystem/OT pos control/adjust_for_heading ==
  original : Inport
  Memory : Memory
  adjust_pitch_command : MATLAB Function  TreatAsAtomicUnit=on
  heading_adjusted pitch : Outport
  wires:
  [heading_obs] -> adjust_pitch_command/3(heading)
  adjust_pitch_command/1(adj_pitch_cmd) -> Memory/1
  [roll_workspace_frame] -> adjust_pitch_command/2(roll_cmd)
  original/1 -> adjust_pitch_command/1(pitch_cmd)
  Memory/1 -> heading_adjusted pitch/1

== system leader_qball2_mytest/Pitch Controller/Subsystem/OT pos control/rate limitted control ==
  error : Inport
  Gain4 : Gain  Gain=-1
  Integrator : Integrator  ExternalReset=level
  Integrator reset : Subsystem
  Ki - Battery DOWN : Gain  Gain=KiOUTER_PITCH_DOWN
  Ki - Battery UP : Gain  Gain=KiOUTER_PITCH_UP
  Kp - Battery DOWN : Gain  Gain=KpOUTER_PITCH_DOWN
  Kp - Battery UP : Gain  Gain=KpOUTER_PITCH_UP
  Kv - Battery DOWN : Gain  Gain=KdOUTER_PITCH_DOWN
  Kv - Battery UP : Gain  Gain=KdOUTER_PITCH_UP
  Saturation1 : Saturate  UpperLimit=LIMIT_CMD_PITCH  LowerLimit=-LIMIT_CMD_PITCH
  Second-Order Low-Pass Filter1 : quarc_library/Continuous/Second-Order Low-Pass Filter  params_source=Internal (dialog parameters)  input_width=OMEGA_DIFF  input_zeta=1  input_init=0
  Sum4 : Sum  Inputs=-++
  Switch - Kd : Switch  Criteria=u2 > Threshold  Threshold=0.5
  Switch - Ki : Switch  Criteria=u2 > Threshold  Threshold=0.5
  Switch - Kp : Switch  Criteria=u2 > Threshold  Threshold=0.5
  Terminator4 : Terminator
  Pitch Ref CMD (rad) : Outport
  wires:
  Gain4/1 -> Pitch Ref CMD (rad)/1
  Saturation1/1 -> Gain4/1
  error/1 -> Kp - Battery UP/1, Ki - Battery UP/1, Ki - Battery DOWN/1, Kp - Battery DOWN/1
  Sum4/1 -> Saturation1/1
  Second-Order Low-Pass Filter1/2 -> Kv - Battery UP/1, Kv - Battery DOWN/1
  Integrator/1 -> Sum4/3
  [z_optitrack] -> Second-Order Low-Pass Filter1/1
  Integrator reset/1(r) -> Integrator/2
  Second-Order Low-Pass Filter1/1 -> Terminator4/1
  Kv - Battery DOWN/1 -> Switch - Kd/3
  Kv - Battery UP/1 -> Switch - Kd/1
  [BatteryOnTop] -> Switch - Kd/2, Switch - Kp/2, Switch - Ki/2
  Switch - Kd/1 -> Sum4/1
  Switch - Kp/1 -> Sum4/2
  Kp - Battery UP/1 -> Switch - Kp/1
  Kp - Battery DOWN/1 -> Switch - Kp/3
  Ki - Battery UP/1 -> Switch - Ki/1
  Ki - Battery DOWN/1 -> Switch - Ki/3
  Switch - Ki/1 -> Integrator/1

== system leader_qball2_mytest/Pitch Controller/Subsystem/Safety - Emergency Landing Zero Ref CMD/Enabled Subsystem ==
  Enable : EnablePort
  Constant : Constant
  Out1 : Outport  InitialOutput=0
  wires:
  Constant/1 -> Out1/1

== system leader_qball2_mytest/Roll Controller/Subsystem/OT pos control/adjust_for_heading ==
  original : Inport
  Memory : Memory
  adjust_roll_command : MATLAB Function  TreatAsAtomicUnit=on
  heading_adjusted roll : Outport
  wires:
  [heading_obs] -> adjust_roll_command/3(heading)
  [pitch_workspace_frame] -> adjust_roll_command/2(pitch_cmd)
  original/1 -> adjust_roll_command/1(roll_cmd)
  adjust_roll_command/1(adj_roll_cmd) -> Memory/1
  Memory/1 -> heading_adjusted roll/1

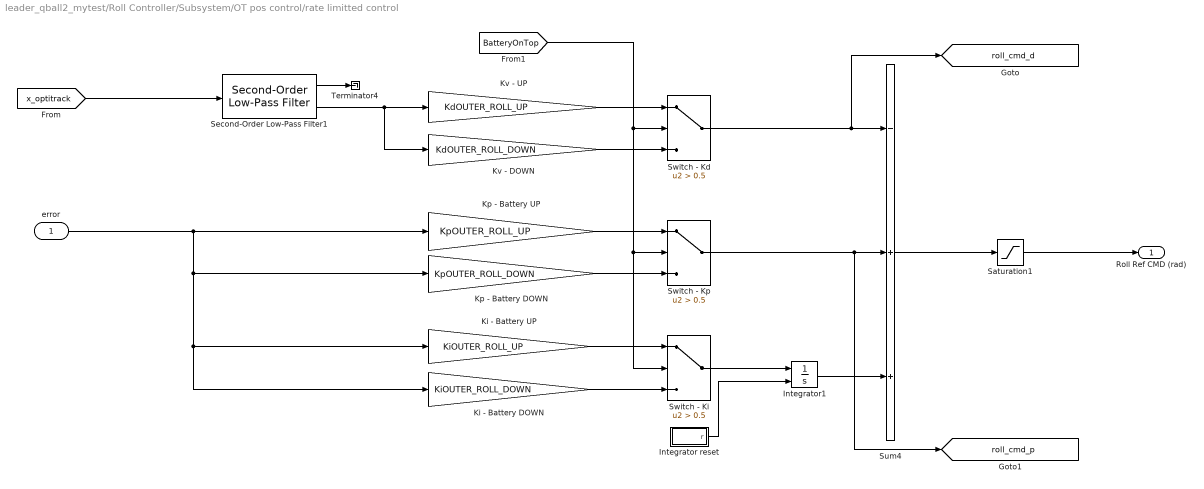
== system leader_qball2_mytest/Roll Controller/Subsystem/OT pos control/rate limitted control ==
  error : Inport
  Integrator reset : Subsystem
  Integrator1 : Integrator  ExternalReset=level
  Ki - Battery DOWN : Gain  Gain=KiOUTER_ROLL_DOWN
  Ki - Battery UP : Gain  Gain=KiOUTER_ROLL_UP
  Kp - Battery DOWN : Gain  Gain=KpOUTER_ROLL_DOWN
  Kp - Battery UP : Gain  Gain=KpOUTER_ROLL_UP
  Kv - DOWN : Gain  Gain=KdOUTER_ROLL_DOWN
  Kv - UP : Gain  Gain=KdOUTER_ROLL_UP
  Saturation1 : Saturate  UpperLimit=LIMIT_CMD_ROLL  LowerLimit=-LIMIT_CMD_ROLL
  Second-Order Low-Pass Filter1 : quarc_library/Continuous/Second-Order Low-Pass Filter  params_source=Internal (dialog parameters)  input_width=OMEGA_DIFF  input_zeta=1  input_init=0
  Sum4 : Sum  Inputs=-++
  Switch - Kd : Switch  Criteria=u2 > Threshold  Threshold=0.5
  Switch - Ki : Switch  Criteria=u2 > Threshold  Threshold=0.5
  Switch - Kp : Switch  Criteria=u2 > Threshold  Threshold=0.5
  Terminator4 : Terminator
  Roll Ref CMD (rad) : Outport
  tag scope: roll_cmd_d=global, roll_cmd_p=global
  wires:
  Saturation1/1 -> Roll Ref CMD (rad)/1
  error/1 -> Kp - Battery UP/1, Ki - Battery UP/1, Ki - Battery DOWN/1, Kp - Battery DOWN/1
  Sum4/1 -> Saturation1/1
  Second-Order Low-Pass Filter1/2 -> Kv - DOWN/1, Kv - UP/1
  Integrator reset/1(r) -> Integrator1/2
  Integrator1/1 -> Sum4/3
  [x_optitrack] -> Second-Order Low-Pass Filter1/1
  Second-Order Low-Pass Filter1/1 -> Terminator4/1
  Kv - UP/1 -> Switch - Kd/1
  Kv - DOWN/1 -> Switch - Kd/3
  Switch - Kd/1 -> [roll_cmd_d], Sum4/1
  Kp - Battery DOWN/1 -> Switch - Kp/3
  Kp - Battery UP/1 -> Switch - Kp/1
  [BatteryOnTop] -> Switch - Kp/2, Switch - Ki/2, Switch - Kd/2
  Switch - Kp/1 -> [roll_cmd_p], Sum4/2
  Ki - Battery UP/1 -> Switch - Ki/1
  Ki - Battery DOWN/1 -> Switch - Ki/3
  Switch - Ki/1 -> Integrator1/1

== system leader_qball2_mytest/Roll Controller/Subsystem/Safety - Emergency Landing Zero Ref CMD/Enabled Subsystem ==
  Enable : EnablePort
  Constant : Constant
  Out1 : Outport  InitialOutput=0
  wires:
  Constant/1 -> Out1/1

== system leader_qball2_mytest/Throttle and height control/Safety - Active During Emergency Landing: Ramp Throttle CMD down to zero if Sonar Failed /Subsystem/Enabled Subsystem1 ==
  timeout limit : Inport
  Enable : EnablePort  StatesWhenEnabling=reset
  Constant : Constant  SampleTime=qc_get_step_size
  Discrete-Time Integrator : DiscreteIntegrator  SampleTime=-1  ICPrevOutput=DiscIntNeverNeededParam  ICPrevScaledInput=DiscIntNeverNeededParam
  Relational Operator : RelationalOperator  OutDataTypeStr=boolean
  timeout : Outport  OutputWhenDisabled=reset  InitialOutput=[0]
  wires:
  Constant/1 -> Discrete-Time Integrator/1
  Discrete-Time Integrator/1 -> Relational Operator/1
  timeout limit/1 -> Relational Operator/2
  Relational Operator/1 -> timeout/1

== system leader_qball2_mytest/Throttle and height control/height control/Safety - Emergency Landing (Set Height Ref CMD to zero)/Enabled Subsystem ==
  Enable : EnablePort
  Constant : Constant
  Out1 : Outport  InitialOutput=0
  wires:
  Constant/1 -> Out1/1

== system leader_qball2_mytest/Throttle and height control/height control/sigmoid1/arm height command ==
  In1 : Inport
  Enable : EnablePort
  Out1 : Outport  OutputWhenDisabled=reset  InitialOutput=0
  wires:
  In1/1 -> Out1/1

== system leader_qball2_mytest/Throttle and height control/height control/sigmoid1/sigmoid limits ==
  note: 0.2
  note: 1
  height cmd : Inport
  height : Inport  Port=2
  Compare To Constant : simulink/Logic and Bit Operations/Compare To Constant  relop=<=  const=0.5  OutDataTypeStr=uint8  ZeroCross=off
  Compare To Constant1 : simulink/Logic and Bit Operations/Compare To Constant  relop=<=  const=0.2  OutDataTypeStr=uint8  ZeroCross=off
  Demux : Demux  Outputs=2
  Logical Operator : Logic  Operator=OR  AllPortsSameDT=off  OutDataTypeStr=boolean
  Mux : Mux  Inputs=2
  Mux1 : Mux  Inputs=2
  Switch : Switch  Threshold=0.5
  amax flight : Constant  Value=10
  amax takeoff : Constant  Value=0.2
  vmax flight : Constant  Value=2
  vmax takeoff : Constant  Value=2
  vmax : Outport
  amax : Outport  Port=2
  wires:
  height/1 -> Compare To Constant/1
  vmax takeoff/1 -> Mux/1
  amax takeoff/1 -> Mux/2
  Mux/1 -> Switch/1
  vmax flight/1 -> Mux1/1
  amax flight/1 -> Mux1/2
  Mux1/1 -> Switch/3
  Switch/1 -> Demux/1
  Demux/1 -> vmax/1
  Demux/2 -> amax/1
  Compare To Constant/1 -> Logical Operator/1
  height cmd/1 -> Compare To Constant1/1
  Compare To Constant1/1 -> Logical Operator/2
  Logical Operator/1 -> Switch/2

== system leader_qball2_mytest/Throttle and height control/height control/sonar controller/Integrator reset ==
  Logical Operator1 : Logic  Operator=NOT  AllPortsSameDT=off  OutDataTypeStr=boolean
  Logical Operator2 : Logic  AllPortsSameDT=off  OutDataTypeStr=boolean
  Memory : Memory  InheritSampleTime=on  LinearizeMemory=on  LinearizeAsDelay=on
  r : Outport
  wires:
  Memory/1 -> Logical Operator2/2
  Logical Operator2/1 -> r/1
  [soft_land] -> Memory/1
  Logical Operator1/1 -> Logical Operator2/1
  [armed] -> Logical Operator1/1

== system leader_qball2_mytest/DAQ/Initialize sensors/Sensor Fusion//Filtering/Signal Conditioning - Sonar/FOH1 ==
  Input : Inport
  Bias : Bias  Bias=-Ts
  Clock : Clock
      settings: DisableCoverage=on
  Digital Clock : DigitalClock  DisableCoverage=on  SampleTime=Ts
  Gain : Gain  DisableCoverage=on  Gain=1/Ts  SaturateOnIntegerOverflow=on  OutDataTypeStr=Inherit: Same as input  ParamDataTypeStr=Inherit: Same as input
  Product : Product  RndMeth=Zero
  Rate Transition : RateTransition
  Rate Transition1 : RateTransition  OutPortSampleTime=qc_get_step_size
  Rate Transition3 : RateTransition  OutPortSampleTime=qc_get_step_size
  Rate Transition4 : RateTransition  OutPortSampleTime=Ts
  Rate Transition5 : RateTransition  OutPortSampleTime=qc_get_step_size
  Scope : Scope
  Scope1 : Scope
      settings: SaveName=ScopeData2
  Sum : Sum  DisableCoverage=on  Inputs=|+-  SaturateOnIntegerOverflow=on  InputSameDT=on  OutDataTypeStr=Inherit: Same as first input
  Sum2 : Sum  DisableCoverage=on  Inputs=|+-  SaturateOnIntegerOverflow=on  InputSameDT=on  OutDataTypeStr=Inherit: Same as first input
  Unit Delay : UnitDelay  DisableCoverage=on  SampleTime=Ts
  s : Sum  Inputs=++|  SaturateOnIntegerOverflow=on  InputSameDT=on  OutDataTypeStr=Inherit: Same as first input
  Output : Outport
  wires:
  Rate Transition4/1 -> Unit Delay/1, Sum/1
  Input/1 -> Rate Transition4/1, Rate Transition5/1
  Unit Delay/1 -> Sum/2
  Rate Transition1/1 -> Product/1, Scope1/1
  Product/1 -> s/2
  Rate Transition3/1 -> Product/2, Scope/1
  Sum/1 -> Rate Transition1/1
  Bias/1 -> Sum2/1
  Clock/1 -> Bias/1
  Rate Transition/1 -> Sum2/2
  s/1 -> Output/1
  Rate Transition5/1 -> s/1
  Gain/1 -> Rate Transition3/1
  Digital Clock/1 -> Rate Transition/1
  Sum2/1 -> Gain/1

== system leader_qball2_mytest/DAQ/Initialize sensors/Sensor Fusion//Filtering/Signal Conditioning - Sonar/Sampler ==
  In1 : Inport
  Derivative : Derivative
  Digital Clock : DigitalClock  DisableCoverage=on  SampleTime=0.1
  Rate Transition : RateTransition
  Triggered Subsystem : Subsystem  TreatAsAtomicUnit=on
  Out1 : Outport
  wires:
  Derivative/1 -> Triggered Subsystem/Trigger
  Rate Transition/1 -> Derivative/1
  Digital Clock/1 -> Rate Transition/1
  In1/1 -> Triggered Subsystem/1(In1)
  Triggered Subsystem/1(Out1) -> Out1/1

== system leader_qball2_mytest/Pitch Controller/Subsystem/OT pos control/rate limitted control/Integrator reset ==
  Logical Operator1 : Logic  Operator=NOT  AllPortsSameDT=off  OutDataTypeStr=boolean
  r : Outport
  wires:
  Logical Operator1/1 -> r/1
  [armed] -> Logical Operator1/1

== system leader_qball2_mytest/Roll Controller/Subsystem/OT pos control/rate limitted control/Integrator reset ==
  Logical Operator1 : Logic  Operator=NOT  AllPortsSameDT=off  OutDataTypeStr=boolean
  r : Outport
  wires:
  Logical Operator1/1 -> r/1
  [armed] -> Logical Operator1/1

== system leader_qball2_mytest/DAQ/Initialize sensors/Sensor Fusion//Filtering/Signal Conditioning - Sonar/Sampler/Triggered Subsystem ==
  In1 : Inport
  Trigger : TriggerPort
  Out1 : Outport
  wires:
  In1/1 -> Out1/1

== matlab function leader_qball2_mytest/Throttle and height control/Joystick mode throttle/Joystick to Throttle Mapping ==
  data: u input; y output; l1 input; l2 input
function y = fcn(u,l1,l2)
% This block supports the Embedded MATLAB subset.
% See the help menu for details. 
% l1 = .6;
% l2 = .9;

if u<.1
    y = 0;%.8/.1*u
else
    y = (l2-l1)/(1-.1)*(u-.1)+l1;
end

== matlab function leader_qball2_mytest/DAQ/Initialize sensors/Sensor Fusion//Filtering/Kalman Filter - Pitch ==
  data: angle output; acc_angle input; gyro_rate input; opti_angle input; dt input; BatteryOnTop input
function angle   = fcn(acc_angle,gyro_rate,opti_angle,dt,BatteryOnTop)
%#eml

    if(BatteryOnTop == 1)
        Q_angle = 0.001; %0.01; %0.001
    else
        Q_angle = 0.01;
    end;
     Q_gyro   = 0.01; %0.01;  %0.003
     R_angle  =  0.03;  %0.03

    
    persistent P_00;
    persistent P_01;
    persistent P_10;
    persistent P_11;
    persistent x_angle;
    persistent x_bias;
        
    if isempty(P_00)
        P_00 = 0;
    end
    
    if isempty(P_01)
        P_01 = 0;
    end
    if isempty(P_10)
        P_10 = 0;
    end
    if isempty(P_11)
        P_11 = 0;
    end
     if isempty(x_bias)
        x_bias = 0;
     end
     if isempty(x_angle)
        x_angle = 0;
     end
    
    
    % Calculate the new output
    x_angle = x_angle + dt * (gyro_rate - x_bias);
    P_00 = P_00 -  dt * (P_10 + P_01) + Q_angle * dt;
    P_01 = P_01  - dt * P_11;
    P_10 = P_10  - dt * P_11;
    P_11 = P_11  + Q_gyro * dt;

    % Assuming H = [0.98 (effect of gyro) 0.02 (effect of acc)]
    %e = (0.97*x_angle + 0.03*acc_angle) - x_angle;
    e = (0.9*x_angle + 0.01*acc_angle+0.09*opti_angle) - x_angle;
    S = P_00 + R_angle;
    K_0 = P_00 / S;
    K_1 = P_10 / S;

    % Correction
    x_angle = x_angle+  K_0 * e;
    x_bias  = x_bias+  K_1 * e;
    P_00 = P_00 - K_0 * P_00;
    P_01 = P_01 - K_0 * P_01;
    P_10 = P_10 - K_1 * P_00;
    P_11 = P_11 - K_1 * P_01;

    angle = x_angle;

== matlab function leader_qball2_mytest/Throttle and height control/height control/sonar controller/User-controller landing state machine ==
  data: cmd input; y output; height input; u input; land output; rate input
function [y, land] = fcn(cmd, height, u, rate)
% This block supports the Embedded MATLAB subset.
% See the help menu for details. 

% state variable
%   0 : landed state. Motors off until cmd > 0.
%   1 : fly state. Motors enabled until cmd <= 0 AND height <= 0.20 m.
persistent state;

% c variable: represents the latched control signal.
persistent c;

if isempty(state)
    state = 0;
end
if isempty(c)
    c = 0;
end

land = 0;

switch state
    case 0
        if cmd > 0
            state = 1;
            c = u;
            y = u;
        else
            land = 1;
            c = c - rate;
            if c < 0
                c = 0;
            end
            y = c;
        end
        
    case 1
        c = u;
        y = u;
        if cmd <= 0 && height <= 0.08
            state = 0;
            land = 1;
        end
        
    otherwise
        y = c;
end

== matlab function leader_qball2_mytest/Throttle and height control/Height joystick adjust/MATLAB Function ==
  data: throttle input; enable output; step_size input
function enable = active_state(throttle,step_size)
%#eml

persistent state;
persistent counter;

if(isempty(state))
    state = 0; % Idle
end;

if(isempty(counter))
    counter = 0; % time delay counter
end;

threshold = 0.2;
timelimit = 3.5/step_size;

switch state
    case 0 % Idle
        enable = 0;
        if( throttle > threshold )
            state = 1;  % armed
        end;
    case 1 % Armed
        enable = 0;
        counter = counter + 1;
        if( counter >= timelimit )
            state = 2;  % Active
            counter = 0;
        end;
        if( throttle < threshold )
            state = 0;
            counter = 0;
        end;
    case 2 % Active
        enable = 1;
        if( throttle < threshold )
            state = 0;
        end;
    otherwise
        enable=0;
        state=0;
        counter=0;
end;

== matlab function leader_qball2_mytest/Data from host/Subsystem4/Embedded MATLAB Function ==
  data: u input; y output; x input; threshold input
function y = fcn(u,x,threshold)
% This block supports the Embedded MATLAB subset.
% See the help menu for details. 

if ((u < threshold) && (u > -threshold))
    y = u;
else
    y = x;
end

== matlab function leader_qball2_mytest/Data from host/Subsystem5/Embedded MATLAB Function ==
  data: u input; y output; x input; threshold input
function y = fcn(u,x,threshold)
% This block supports the Embedded MATLAB subset.
% See the help menu for details. 

if ((u < threshold) && (u > -threshold))
    y = u;
else
    y = x;
end

== matlab function leader_qball2_mytest/Data from host/Subsystem6/Embedded MATLAB Function ==
  data: u input; y output; x input; threshold input
function y = fcn(u,x,threshold)
% This block supports the Embedded MATLAB subset.
% See the help menu for details. 

if ((u < threshold) && (u > -threshold))
    y = u;
else
    y = x;
end
